simulink model "Project3"  (R2021a)
settings: Solver=FixedStepDiscrete  StartTime=0.0  StopTime=55  RelTol=1e-3
libraries: hdlBasic x25, xbsIndex_r4 x1
settings Model: Creator=cavallar  LastModifiedBy=user
settings SolverCC: AlgebraicLoopSolver=TrustRegion
settings DataIOCC: LimitDataPoints=on  SaveFormat=Array  ReturnWorkspaceOutputs=off
settings OptimizationCC: LifeSpan=inf
settings DebuggingCC: SFUnexpectedBacktrackingDiag=warning  SFNoUnconditionalDefaultTransitionDiag=warning  SFExecutionAtInitializationDiag=none  SFMachineParentedDataDiag=warning  ArithmeticOperatorsInVariantConditions=warning
settings HardwareCC: ProdBitPerPointer=32  ProdBitPerSizeT=32  ProdBitPerPtrDiffT=32  ProdLargestAtomicFloat=None  ProdIntDivRoundTo=Undefined  ProdEndianess=Unspecified  ProdWordSize=32  ProdHWDeviceType=32-bit Generic
settings ModelReferenceCC: PropagateSignalLabelsOutOfModel=off
settings SFSimCC: SimUseLocalCustomCode=off  CustomCodeUndefinedFunction=UseInterfaceOnly
settings RTWCC: RTWUseLocalCustomCode=off
settings CodeAppCC: StateflowObjectComments=on
settings GRTTargetCC: TargetLangStandard=C89/C90 (ANSI)
settings ConfigComp: CovMetricSettings=dw  CovSaveCumulativeToWorkspaceVar=on  CovSaveSingleToWorkspaceVar=on  CovExternalEMLEnable=off  CovSFcnEnable=off

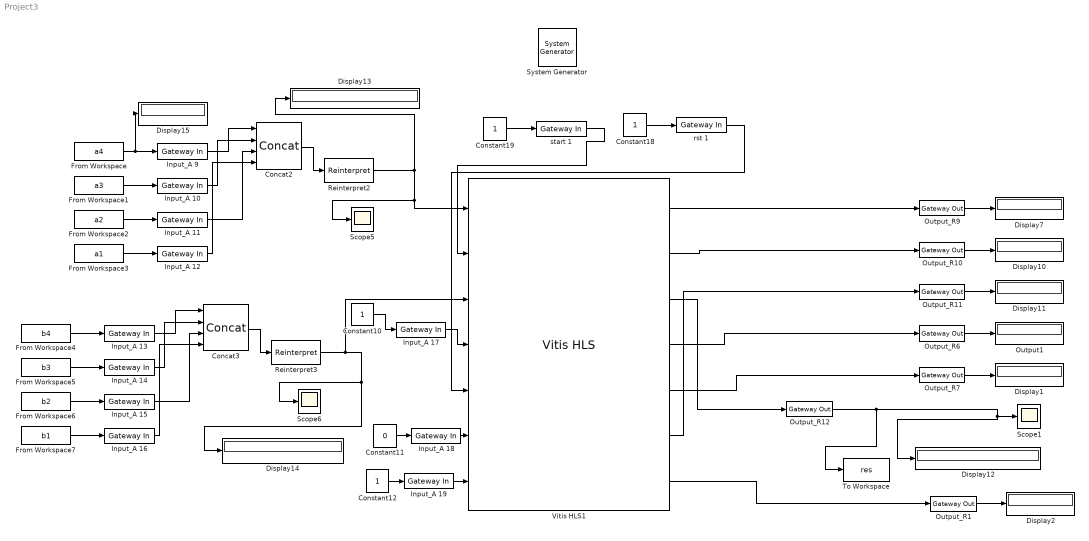
== system Project3 ==
  " System Generator" : xbsIndex_r4/ System Generator  Tag=genX  xilinxfamily=zynq  part=xc7z020  speed=-1  package=clg484  synthesis_tool=Vivado  clock_wrapper=Clock Enables  directory=C:/ELEC522/am251/proj3/netlist  proj_type=Vivado  Synth_file=Vivado Synthesis Defaults  Impl_file=Vivado Implementation Defaults  testbench=off  simulink_period=1  sysclk_period=5  dcm_input_clock_period=10  incr_netlist=off  trim_vbits=Everywhere in SubSystem  dbl_ovrd=According to Block Masks  core_generation=According to Block Masks  run_coregen=off  deprecated_control=off  eval_field=0  block_type=sysgen
  Concat2 : hdlBasic/Concat  num_inputs=4  XmcBlockStatus=1  maskContainerNames=group1  block_type=concat  block_config=sysgen:Concat_config
  Concat3 : hdlBasic/Concat  num_inputs=4  XmcBlockStatus=1  maskContainerNames=group1  block_type=concat  block_config=sysgen:Concat_config
  Constant{10,12,18..19} (4 alike) : Constant
  Constant11 : Constant  Value=0
  Display{1..2,7,10..15} (9 alike) : Display
      Display12 settings: Format=hex (Stored Integer)
      Display13 settings: Format=hex (Stored Integer)
      Display14 settings: Format=hex (Stored Integer)
  From Workspace : FromWorkspace  VariableName=a4
  From Workspace1 : FromWorkspace  VariableName=a3
  From Workspace2 : FromWorkspace  VariableName=a2
  From Workspace3 : FromWorkspace  VariableName=a1
  From Workspace4 : FromWorkspace  VariableName=b4
  From Workspace5 : FromWorkspace  VariableName=b3
  From Workspace6 : FromWorkspace  VariableName=b2
  From Workspace7 : FromWorkspace  VariableName=b1
  Input_A {9..16} (8 alike) : hdlBasic/Gateway In  gui_display_data_type=Fixed-point  arith_type=Unsigned  n_bits=16  bin_pt=0  preci_type=Single  exp_width=8  frac_width=24  rows=1  columns=1  quantization="Round  (unbiased: +/- Inf)"  overflow=Saturate  period=1  UseAsADC=off  ADCChannel='1'  interface=None  automatic_assignment=on  address_offset=hex2dec('00')  intf_name=''  intf_description='Input_A'  default_value=0  timing_constraint=None  locs_specified=off  LOCs={}  io_standard={}  inherit_from_input=off  hdl_port=on  XmcBlockStatus=1  maskContainerNames=group4  block_type=gatewayin  block_config=sysgen:gateway_in_config  block_width_w=590  block_height_w=620  block_width=640  block_height=850
  Input_A 17 : hdlBasic/Gateway In  gui_display_data_type=Boolean  arith_type=Boolean  n_bits=16  bin_pt=0  preci_type=Single  exp_width=8  frac_width=24  rows=1  columns=1  quantization="Round  (unbiased: +/- Inf)"  overflow=Saturate  period=1  UseAsADC=off  ADCChannel='1'  interface=None  automatic_assignment=on  address_offset=hex2dec('00')  intf_name=''  intf_description='Input_A'  default_value=0  timing_constraint=None  locs_specified=off  LOCs={}  io_standard={}  inherit_from_input=off  hdl_port=on  XmcBlockStatus=1  maskContainerNames=group4  block_type=gatewayin  block_config=sysgen:gateway_in_config  block_width_w=590  block_height_w=620  block_width=640  block_height=850
  Input_A 18 : hdlBasic/Gateway In  gui_display_data_type=Boolean  arith_type=Boolean  n_bits=16  bin_pt=0  preci_type=Single  exp_width=8  frac_width=24  rows=1  columns=1  quantization="Round  (unbiased: +/- Inf)"  overflow=Saturate  period=1  UseAsADC=off  ADCChannel='1'  interface=None  automatic_assignment=on  address_offset=hex2dec('00')  intf_name=''  intf_description='Input_A'  default_value=0  timing_constraint=None  locs_specified=off  LOCs={}  io_standard={}  inherit_from_input=off  hdl_port=on  XmcBlockStatus=1  maskContainerNames=group4  block_type=gatewayin  block_config=sysgen:gateway_in_config  block_width_w=590  block_height_w=620  block_width=640  block_height=850
  Input_A 19 : hdlBasic/Gateway In  gui_display_data_type=Boolean  arith_type=Boolean  n_bits=16  bin_pt=0  preci_type=Single  exp_width=8  frac_width=24  rows=1  columns=1  quantization="Round  (unbiased: +/- Inf)"  overflow=Saturate  period=1  UseAsADC=off  ADCChannel='1'  interface=None  automatic_assignment=on  address_offset=hex2dec('00')  intf_name=''  intf_description='Input_A'  default_value=0  timing_constraint=None  locs_specified=off  LOCs={}  io_standard={}  inherit_from_input=off  hdl_port=on  XmcBlockStatus=1  maskContainerNames=group4  block_type=gatewayin  block_config=sysgen:gateway_in_config  block_width_w=590  block_height_w=620  block_width=640  block_height=850
  Output1 : Display
  Output_R{1,6..7,9..12} (7 alike) : hdlBasic/Gateway Out  inherit_from_input=on  hdl_port=on  rows=1  columns=1  UseAsDAC=off  DACChannel='1'  interface=None  automatic_assignment=on  address_offset=hex2dec('00')  intf_name=''  intf_description='Output_R'  timing_constraint=None  locs_specified=off  LOCs={}  io_standard={}  XmcBlockStatus=1  maskContainerNames=group4  block_type=gatewayout  block_config=sysgen:gateway_out_config  block_width_w=590  block_height_w=620  block_width=620  block_height=750
  Reinterpret2 : hdlBasic/Reinterpret  force_arith_type=on  arith_type="Signed  (2's comp)"  force_bin_pt=off  bin_pt=0  XmcBlockStatus=1  maskContainerNames=group1  block_type=reinterpret  block_config=sysgen:Reinterpret_config
  Reinterpret3 : hdlBasic/Reinterpret  force_arith_type=on  arith_type="Signed  (2's comp)"  force_bin_pt=off  bin_pt=0  XmcBlockStatus=1  maskContainerNames=group1  block_type=reinterpret  block_config=sysgen:Reinterpret_config
  Scope1 : Scope
  Scope5 : Scope
  Scope6 : Scope
  To Workspace : ToWorkspace  VariableName=res  SaveFormat=Timeseries  SampleTime=-1
      settings: Save2DSignal=2-D array (concatenate along first dimension)
  Vitis HLS1 : hdlBasic/Vitis HLS  anytable='F:\VLSI\am251\project3\lab1project3\lab1project3\solution7'  fast_sim=off  display_datatype=on  rate_propagation_method=Simulink system period  model_file_path=''  latency=1  block_type=vitis_hls
      settings: infoedit=This block allows including C,C++ and SystemC source files in System Generator for DSP designs.
  rst 1 : hdlBasic/Gateway In  gui_display_data_type=Boolean  arith_type=Boolean  n_bits=16  bin_pt=0  preci_type=Single  exp_width=8  frac_width=24  rows=1  columns=1  quantization="Round  (unbiased: +/- Inf)"  overflow=Saturate  period=1  UseAsADC=off  ADCChannel='1'  interface=None  automatic_assignment=on  address_offset=hex2dec('00')  intf_name=''  intf_description='Input_A'  default_value=0  timing_constraint=None  locs_specified=off  LOCs={}  io_standard={}  inherit_from_input=off  hdl_port=on  XmcBlockStatus=1  maskContainerNames=group4  block_type=gatewayin  block_config=sysgen:gateway_in_config  block_width_w=590  block_height_w=620  block_width=640  block_height=850
  start 1 : hdlBasic/Gateway In  gui_display_data_type=Boolean  arith_type=Boolean  n_bits=16  bin_pt=0  preci_type=Single  exp_width=8  frac_width=24  rows=1  columns=1  quantization="Round  (unbiased: +/- Inf)"  overflow=Saturate  period=1  UseAsADC=off  ADCChannel='1'  interface=None  automatic_assignment=on  address_offset=hex2dec('00')  intf_name=''  intf_description='Input_A'  default_value=0  timing_constraint=None  locs_specified=off  LOCs={}  io_standard={}  inherit_from_input=off  hdl_port=on  XmcBlockStatus=1  maskContainerNames=group4  block_type=gatewayin  block_config=sysgen:gateway_in_config  block_width_w=590  block_height_w=620  block_width=640  block_height=850
  wires:
  Concat2/1 -> Reinterpret2/1
  Output_R7/1 -> Display1/1
  Input_A 14/1 -> Concat3/2
  Reinterpret3/1 -> Vitis HLS1/3, Display14/1, Scope6/1
  Concat3/1 -> Reinterpret3/1
  Output_R11/1 -> Display11/1
  Input_A 13/1 -> Concat3/1
  From Workspace6/1 -> Input_A 15/1
  Input_A 15/1 -> Concat3/3
  Input_A 9/1 -> Concat2/1
  From Workspace7/1 -> Input_A 16/1
  Vitis HLS1/4 -> Output_R6/1
  Output_R6/1 -> Output1/1
  Input_A 11/1 -> Concat2/3
  Constant19/1 -> start 1/1
  From Workspace3/1 -> Input_A 12/1
  From Workspace5/1 -> Input_A 14/1
  Vitis HLS1/1 -> Output_R9/1
  Input_A 16/1 -> Concat3/4
  Reinterpret2/1 -> Vitis HLS1/1, Scope5/1, Display13/1
  From Workspace4/1 -> Input_A 13/1
  Output_R12/1 -> To Workspace/1, Display12/1, Scope1/1
  From Workspace/1 -> Display15/1, Input_A 9/1
  Constant18/1 -> rst 1/1
  Output_R9/1 -> Display7/1
  Vitis HLS1/2 -> Output_R10/1
  Input_A 12/1 -> Concat2/4
  start 1/1 -> Vitis HLS1/2
  Output_R10/1 -> Display10/1
  Input_A 10/1 -> Concat2/2
  From Workspace1/1 -> Input_A 10/1
  From Workspace2/1 -> Input_A 11/1
  Vitis HLS1/5 -> Output_R7/1
  Constant10/1 -> Input_A 17/1
  Input_A 17/1 -> Vitis HLS1/4
  Input_A 18/1 -> Vitis HLS1/6
  Constant11/1 -> Input_A 18/1
  Input_A 19/1 -> Vitis HLS1/7
  Constant12/1 -> Input_A 19/1
  Output_R1/1 -> Display2/1
  Vitis HLS1/7 -> Output_R1/1
  rst 1/1 -> Vitis HLS1/5
  Vitis HLS1/3 -> Output_R12/1
  Vitis HLS1/6 -> Output_R11/1
